simulink model "etc_mask4"  (R2018a)
settings: Solver=FixedStepDiscrete  StartTime=0.0  StopTime=20.0  FixedStep=.01  RelTol=1e-3  EnableMultiTasking=on
PreLoadFcn:
  | etc_controller_data;
Description:
  | This is my help
settings Model: ParamWorkspaceSource=ReferencedWorkspace  Creator=nicholas  LastModifiedBy=bneiswan
settings DataIOCC: LimitDataPoints=on  SaveFormat=Array  SignalLoggingName=sigsOut
settings OptimizationCC: DefaultParameterBehavior=Inlined  ExpressionDepthLimit=2147483647  InitFltsAndDblsToZero=on  LifeSpan=inf
settings DebuggingCC: SaveWithParameterizedLinksMsg=none  UnderspecifiedInitializationDetection=Classic  MergeDetectMultiDrivingBlocksExec=none  MultiTaskDSMMsg=warning  MultiTaskCondExecSysMsg=none  ParameterPrecisionLossMsg=none  FcnCallInpInsideContextMsg=warning  AllowSymbolicDim=off  StateNameClashWarn=warning  SFUnexpectedBacktrackingDiag=warning  SFNoUnconditionalDefaultTransitionDiag=warning  SFExecutionAtInitializationDiag=none
settings HardwareCC: ProdBitPerPointer=32  ProdBitPerSizeT=32  ProdBitPerPtrDiffT=32  ProdLargestAtomicFloat=None  ProdIntDivRoundTo=Undefined  ProdEndianess=Unspecified  ProdWordSize=32  ProdHWDeviceType=32-bit Generic  TargetIntDivRoundTo=Zero  TargetEndianess=BigEndian  TargetHWDeviceType=Motorola PowerPC
settings ModelReferenceCC: PropagateSignalLabelsOutOfModel=off
settings CodeAppCC: StateflowObjectComments=on
settings GRTTargetCC: TargetFcnLib=ansi_tfl_tmw.mat  TargetLangStandard=C89/C90 (ANSI)  GeneratePreprocessorConditionals=Disable all  CombineOutputUpdateFcns=off  GRTInterface=on
settings ConfigComp: CovMetricSettings=dw  CovHtmlReporting=on  CovSaveCumulativeToWorkspaceVar=on  CovSaveSingleToWorkspaceVar=on  CovExternalEMLEnable=off  CovSFcnEnable=off

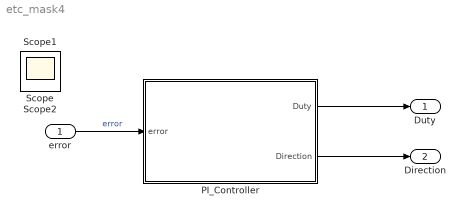
== system etc_mask4 ==
  error : Inport
  PI_Controller : Subsystem  mask(PI Controller){Kp=0.3, Ki=2, Ts=0.01}
      mask prompts: Kp "Proportional Gain (Kp)"; Ki "Integral Gain (Ki)"; Ts "Sample Time (Ts)"
      mask help:
      | This system implements the dynamics of a discrete PI controller with a rate limiter on the integrator.
      | You must specify the proportional gain (Kp), integral gain (Ki), and sample time (Ts) for the system.
      mask init:
      | str1 = ['Kp = ',num2str(Kp)];
      | str2 = ['Ki = ',num2str(Ki)];
      | str3 = ['Ts = ',num2str(Ts)];
      | label = char(str1,str2,str3);
      mask Help:
      | This system implements the dynamics of a discrete PI controller with a rate limiter on the integrator.
      | The equations for the system are:  <br /><br />
      | 
      | <b>Y(k) = Yp(k) + Yi(k)</b><br />
      | Yp(k) = Kp*e(k)<br />
      | Yi(k) = Yi(k-1) + Ki*Ts*e(k)<br />
      | -1 < Yi(k) < 1<br /><br />
      | 
      | Define values for Kp, Ki, and Ts for this system.
      mask Display: disp(label)
  Duty : Outport
  Direction : Outport  Port=2
  Scope : Scope
  Scope1 : Scope
  Scope2 : Scope
  wires:
  error/1 -> PI_Controller/1(error)  "error"
  PI_Controller/1(Duty) -> Duty/1
  PI_Controller/2(Direction) -> Direction/1

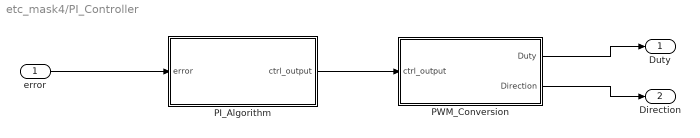
== system etc_mask4/PI_Controller ==
  error : Inport  SampleTime=Ts
  PI_Algorithm : Subsystem
  PWM_Conversion : Subsystem
  Duty : Outport
  Direction : Outport  Port=2
  wires:
  error/1 -> PI_Algorithm/1(error)
  PWM_Conversion/1("Duty ") -> Duty/1
  PWM_Conversion/2(Direction) -> Direction/1
  PI_Algorithm/1(ctrl_output) -> PWM_Conversion/1(ctrl_output)

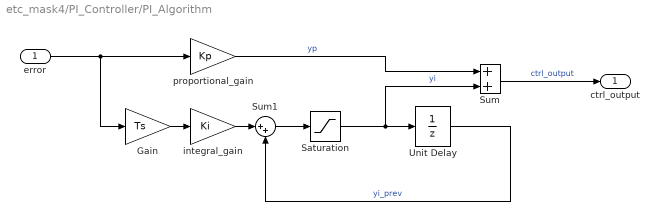
== system etc_mask4/PI_Controller/PI_Algorithm ==
  error : Inport  SampleTime=Ts
      settings: AttributesFormatString=Sample time = %<SampleTime>
  Gain : Gain  Gain=Ts  SaturateOnIntegerOverflow=on  OutDataTypeStr=Inherit: Same as input  ParamDataTypeStr=Inherit: Same as input
  Saturation : Saturate  UpperLimit=1  LowerLimit=-1
      settings: AttributesFormatString=Max: %<UpperLimit>\nMin: %<LowerLimit>
  Sum : Sum  SaturateOnIntegerOverflow=on  InputSameDT=on  OutDataTypeStr=Inherit: Same as first input
  Sum1 : Sum  Inputs=|++  SaturateOnIntegerOverflow=on  InputSameDT=on  OutDataTypeStr=Inherit: Same as first input
  Unit Delay : UnitDelay  SampleTime=Ts
      settings: AttributesFormatString=yi0 = %<X0>\nSample time = %<SampleTime>
  integral_gain : Gain  Gain=Ki  SaturateOnIntegerOverflow=on  OutDataTypeStr=Inherit: Same as input  ParamDataTypeStr=Inherit: Same as input
  proportional_gain : Gain  Gain=Kp  SaturateOnIntegerOverflow=on  OutDataTypeStr=Inherit: Same as input  ParamDataTypeStr=Inherit: Same as input
  ctrl_output : Outport
  wires:
  proportional_gain/1 -> Sum/1  "yp"
  integral_gain/1 -> Sum1/1
  Gain/1 -> integral_gain/1
  Unit Delay/1 -> Sum1/2  "yi_prev"
  Sum1/1 -> Saturation/1
  Saturation/1 -> Unit Delay/1, Sum/2  "yi"
  error/1 -> proportional_gain/1, Gain/1
  Sum/1 -> ctrl_output/1  "ctrl_output"

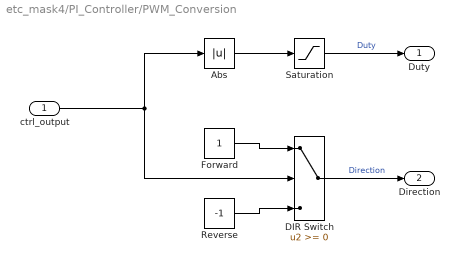
== system etc_mask4/PI_Controller/PWM_Conversion ==
  ctrl_output : Inport
  Abs : Abs
  DIR Switch : Switch
      settings: AttributesFormatString=Criteria: %<Criteria>\nThreshold: %<Threshold>
  Forward : Constant  OutDataTypeStr=double
  Reverse : Constant  Value=-1  OutDataTypeStr=double
  Saturation : Saturate  UpperLimit=1  LowerLimit=0
      settings: AttributesFormatString=%<LowerLimit> < duty < %<UpperLimit>
  "Duty " : Outport
  Direction : Outport  Port=2
  wires:
  Abs/1 -> Saturation/1
  Saturation/1 -> "Duty "/1  "Duty"
  DIR Switch/1 -> Direction/1  "Direction"
  Reverse/1 -> DIR Switch/3
  Forward/1 -> DIR Switch/1
  ctrl_output/1 -> DIR Switch/2, Abs/1
